simulink model "sampleModel56"  (Simulink 9.1)
settings: Solver=VariableStepAuto  StartTime=0.0  StopTime=10.0  RelTol=1e-3
undefined symbols (not defined in the file): DiscIntNeverNeededParam, Newton, Raphson
libraries: simulink x48
(part 1 of 2)
settings Model: SuppressorTable="22 serialization::archive 11 0 6 0 0 2 8 0 0 0 0 6 0 0 1 0 21 sampleModel56/cfblk75 0 6 0 0 2 8 0 0 0 0 6 41 Simulink:DataType:WarningOverFlowDetected 0 0 0 6 0  0  0 0 0 0 8 20160523 0 0 0 10 57 55 0 1 40 SimulinkFixedPoint:util:Overflowoccurred 0 0 0  0  8 20160523 0 10 57 55 0 1 1 0 21 sampleModel56/cfblk69 2 8 0 41 Simulink:DataType:WarningOverFlowDetected 0 0 0  0  8 20160608 0 15 23 17 0 1 40 SimulinkFixedPoint:util:Overflowoccurred 0 0 0  0  8 20160608 0 15 23 17 0 1"  Creator=DELL  LastModifiedBy=DELL
settings DataIOCC: SaveFormat=Dataset
settings OptimizationCC: LifeSpan=auto
settings DebuggingCC: UnderspecifiedInitializationDetection=Simplified  MergeDetectMultiDrivingBlocksExec=error  SFUnexpectedBacktrackingDiag=error  SFNoUnconditionalDefaultTransitionDiag=error  SFExecutionAtInitializationDiag=warning
settings HardwareCC: ProdBitPerPointer=64  ProdBitPerSizeT=64  ProdBitPerPtrDiffT=64  ProdLargestAtomicFloat=Float  ProdIntDivRoundTo=Zero  ProdEndianess=LittleEndian  ProdWordSize=64  ProdHWDeviceType=Intel->x86-64 (Windows64)
settings ModelReferenceCC: PropagateSignalLabelsOutOfModel=on
settings CodeAppCC: StateflowObjectComments=off
settings GRTTargetCC: TargetLangStandard=C99 (ISO)  CombineOutputUpdateFcns=on  GRTInterface=off
settings ConfigComp: CovMetricSettings=dwe  CovHtmlReporting=off  CovSaveCumulativeToWorkspaceVar=off  CovSaveSingleToWorkspaceVar=off  CovExternalEMLEnable=on

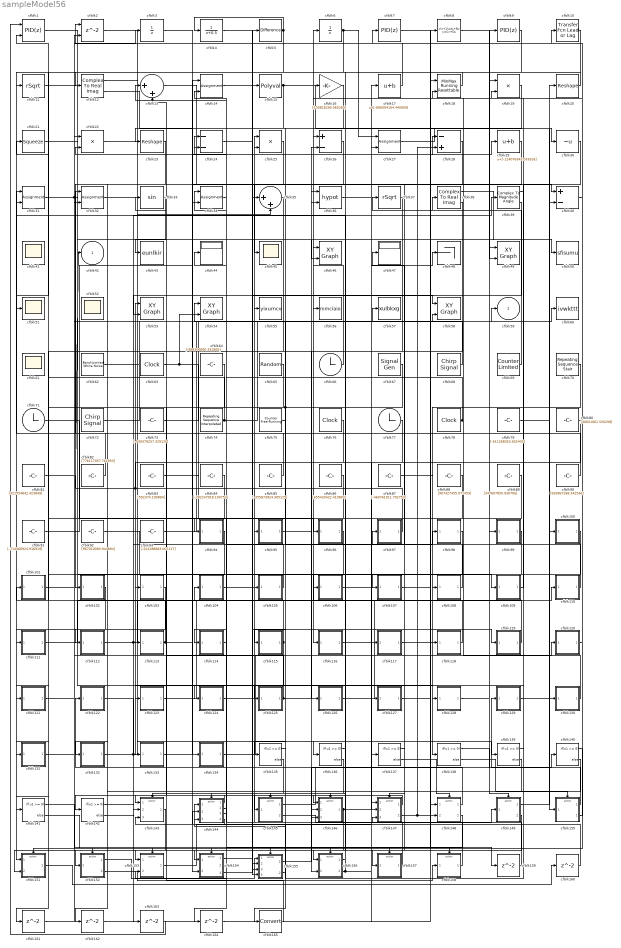
== system sampleModel56 ==
  cfblk1 : simulink/Continuous/PID Controller (2DOF)  Controller=PID  TimeDomain=Discrete-time  SampleTime=1  IntegratorMethod=Forward Euler  FilterMethod=Forward Euler  Form=Parallel  UseFilter=on  ControllerParametersSource=internal  P=1  I=1  D=0  N=100  b=1  c=1  InitialConditionSource=internal  InitialConditionForIntegrator=0  InitialConditionForFilter=0  ExternalReset=none  LimitOutput=off  UpperSaturationLimit=inf  LowerSaturationLimit=-inf  LinearizeAsGain=off  AntiWindupMode=none  Kb=1  TrackingMode=off  Kt=1  PParamMin=[]  PParamMax=[]  IParamMin=[]  IParamMax=[]  DParamMin=[]  DParamMax=[]  NParamMin=[]  NParamMax=[]  bParamMin=[]  bParamMax=[]  cParamMin=[]  cParamMax=[]  KbParamMin=[]  KbParamMax=[]  KtParamMin=[]  KtParamMax=[]  POutMin=[]  POutMax=[]  IOutMin=[]  IOutMax=[]  DOutMin=[]  DOutMax=[]  NOutMin=[]  NOutMax=[]  bOutMin=[]  bOutMax=[]  cOutMin=[]  cOutMax=[]  KbOutMin=[]  KbOutMax=[]  KtOutMin=[]  KtOutMax=[]  IntegratorOutMin=[]  IntegratorOutMax=[]  FilterOutMin=[]  FilterOutMax=[]  SumOutMin=[]  SumOutMax=[]  Sum1OutMin=[]  Sum1OutMax=[]  Sum2OutMin=[]  Sum2OutMax=[]  Sum3OutMin=[]  Sum3OutMax=[]  SumI1OutMin=[]  SumI1OutMax=[]  SumI2OutMin=[]  SumI2OutMax=[]  SumI3OutMin=[]  SumI3OutMax=[]  SumDOutMin=[]  SumDOutMax=[]  SaturationOutMin=[]  SaturationOutMax=[]  IntegratorContinuousStateAttributes=''  IntegratorStateMustResolveToSignalObject=off  IntegratorRTWStateStorageClass=Auto  FilterContinuousStateAttributes=''  FilterStateMustResolveToSignalObject=off  FilterRTWStateStorageClass=Auto  DifferentiatorICPrevScaledInput=0  DifferentiatorOutMin=[]  DifferentiatorOutMax=[]  FilterDiffOutCoefMin=[]  FilterDiffOutCoefMax=[]  SumDenOutMin=[]  SumDenOutMax=[]  SumNumOutMin=[]  SumNumOutMax=[]  ReciprocalOutMin=[]  ReciprocalOutMax=[]  DivideOutMin=[]  DivideOutMax=[]  TunerSelectOption=Transfer Function Based (PID Tuner App)
  cfblk10 : simulink/Discrete/Transfer Fcn Lead or Lag  PoleZ=0.95  ZeroZ=0.75  ICPrevOutput=0.0  ICPrevInput=0.0  DoSatur=off
      settings: SourceProductName=Simulink  SourceProductBaseCode=SL
  cfblk100 : Subsystem
  cfblk101 : Subsystem
  cfblk102 : Subsystem
  cfblk103 : Subsystem
  cfblk104 : Subsystem
  cfblk105 : Subsystem
  cfblk106 : Subsystem
  cfblk107 : Subsystem
  cfblk108 : Subsystem
  cfblk109 : Subsystem
  cfblk11 : Sqrt  Operator=rSqrt  AlgorithmType=Newton-Raphson  SaturateOnIntegerOverflow=on
  cfblk110 : Subsystem
  cfblk111 : Subsystem
  cfblk112 : Subsystem
  cfblk113 : Subsystem
  cfblk114 : Subsystem
  cfblk115 : Subsystem
  cfblk116 : Subsystem
  cfblk117 : Subsystem
  cfblk118 : Subsystem
  cfblk119 : Subsystem
  cfblk12 : ComplexToRealImag
  cfblk120 : Subsystem
  cfblk121 : Subsystem
  cfblk122 : Subsystem
  cfblk123 : Subsystem
  cfblk124 : Subsystem
  cfblk125 : Subsystem
  cfblk126 : Subsystem
  cfblk127 : Subsystem
  cfblk128 : Subsystem
  cfblk129 : Subsystem
  cfblk13 : Sum  Inputs=|++
  cfblk130 : Subsystem
  cfblk131 : Subsystem
  cfblk132 : Subsystem
  cfblk133 : Subsystem
  cfblk134 : Subsystem
  cfblk{135..142} (8 alike) : If  IfExpression=u1 >= 0  SampleTime=1
  cfblk{14,27,31..32,34} (5 alike) : Assignment  DiagnosticForDimensions=Warning  IndexOptions=Index vector (dialog)  Indices=1  OutputSizes=1
  cfblk143 : Subsystem  TreatAsAtomicUnit=on
  cfblk144 : Subsystem  TreatAsAtomicUnit=on
  cfblk145 : Subsystem  TreatAsAtomicUnit=on
  cfblk146 : Subsystem  TreatAsAtomicUnit=on
  cfblk147 : Subsystem  TreatAsAtomicUnit=on
  cfblk148 : Subsystem  TreatAsAtomicUnit=on
  cfblk149 : Subsystem  TreatAsAtomicUnit=on
  cfblk15 : Polyval  Coefs=[ +2.081618890e-019, -1.441693666e-014, +4.719686976e-010, -8.536869453e-006, +1.621573104e-001, -8.087801117e+001 ]
  cfblk150 : Subsystem  TreatAsAtomicUnit=on
  cfblk151 : Subsystem  TreatAsAtomicUnit=on
  cfblk152 : Subsystem  TreatAsAtomicUnit=on
  cfblk153 : Subsystem  TreatAsAtomicUnit=on
  cfblk154 : Subsystem  TreatAsAtomicUnit=on
  cfblk155 : Subsystem  TreatAsAtomicUnit=on
  cfblk156 : Subsystem  TreatAsAtomicUnit=on
  cfblk157 : Subsystem  TreatAsAtomicUnit=on
  cfblk158 : Subsystem  TreatAsAtomicUnit=on
  cfblk{159..164} (6 alike) : Delay  SampleTime=1
  cfblk16 : Gain  Gain=[130818295.065280]
  cfblk165 : DataTypeConversion
  cfblk17 : Bias  Bias=[-890094164.440905]
  cfblk18 : simulink/Math Operations/MinMax Running Resettable  Function=min  vinit=0.0
  cfblk19 : Product
  cfblk2 : Delay  ShowEnablePort=on  SampleTime=1
      settings: InputPortMap=u0,e6
  cfblk20 : Reshape
  cfblk21 : Squeeze
  cfblk22 : Product  Inputs=**
  cfblk23 : Reshape
  cfblk24 : Sum  Inputs=--
  cfblk25 : Product  Inputs=**
  cfblk26 : Sum  Inputs=+-
  cfblk28 : Sum  Inputs=-+
  cfblk29 : Bias  Bias=[-124076343.033326]
  cfblk3 : UnitDelay
  cfblk30 : UnaryMinus
  cfblk33 : Trigonometry
  cfblk35 : Sum  Inputs=|++
  cfblk36 : Math  Operator=hypot  SaturateOnIntegerOverflow=on
  cfblk37 : Sqrt  Operator=rSqrt  AlgorithmType=Newton-Raphson  SaturateOnIntegerOverflow=on
  cfblk38 : ComplexToRealImag
  cfblk39 : ComplexToMagnitudeAngle
  cfblk4 : DiscreteTransferFcn  SampleTime=1
  cfblk40 : Sum  Inputs=+-
  cfblk{41,45,51..52,61} (5 alike) : Scope
      cfblk41 settings: Floating=on
      cfblk52 settings: Floating=on
      cfblk61 settings: Floating=on
  cfblk43 : ToWorkspace  VariableName=eunlkir  SaveFormat=Timeseries  SampleTime=-1
  cfblk44 : Display
  cfblk{46,49,53..54,58} (5 alike) : simulink/Sinks/XY Graph  xmin=-1  xmax=1  ymin=-1  ymax=1  st=-1
  cfblk47 : Display
  cfblk48 : Terminator
  cfblk5 : simulink/Discrete/Difference  ICPrevInput=0.0  OutMin=[]  OutMax=[]  OutDataTypeStr=Inherit: Inherit via back propagation  OutDataType=fixdt(1, 16)  OutScaling=2^-10  DoSatur=off
  cfblk50 : ToWorkspace  VariableName=sfisumu  SaveFormat=Timeseries  SampleTime=-1
  cfblk55 : ToWorkspace  VariableName=yixumcv  SaveFormat=Timeseries  SampleTime=-1
  cfblk56 : ToWorkspace  VariableName=mmciaio  SaveFormat=Timeseries  SampleTime=-1
  cfblk57 : ToWorkspace  VariableName=xulbkxg  SaveFormat=Timeseries  SampleTime=-1
  cfblk6 : UnitDelay
  cfblk60 : ToWorkspace  VariableName=ivwkttt  SaveFormat=Timeseries  SampleTime=-1
  cfblk62 : simulink/Sources/Band-Limited White Noise  Cov=[1765669451.498084]  Ts=0.1  seed=[9360864927.000000]
  cfblk63 : DigitalClock
  cfblk64 : Constant  Value=[-898306890.331865]  SampleTime=1
  cfblk65 : UniformRandomNumber  Minimum=[-2929177195.008087]  Maximum=[2486126280.985762]  Seed=[75996113.000000]  SampleTime=0.1
  cfblk66 : Clock
  cfblk67 : SignalGenerator  WaveForm=square  Amplitude=[871101075.158705]
  cfblk68 : simulink/Sources/Chirp Signal  f1=[-436006107.208133]  T=[-770383043.946067]  f2=[-712322538.075546]
  cfblk69 : simulink/Sources/Counter Limited  uplimit=[311.000000]  tsamp=-1
  cfblk7 : simulink/Continuous/PID Controller  Controller=PID  TimeDomain=Discrete-time  SampleTime=1  IntegratorMethod=Forward Euler  FilterMethod=Forward Euler  Form=Parallel  UseFilter=on  ControllerParametersSource=internal  P=1  I=1  D=0  N=100  InitialConditionSource=internal  InitialConditionForIntegrator=0  InitialConditionForFilter=0  ExternalReset=none  LimitOutput=off  UpperSaturationLimit=inf  LowerSaturationLimit=-inf  LinearizeAsGain=off  AntiWindupMode=none  Kb=1  TrackingMode=off  Kt=1  PParamMin=[]  PParamMax=[]  IParamMin=[]  IParamMax=[]  DParamMin=[]  DParamMax=[]  NParamMin=[]  NParamMax=[]  KbParamMin=[]  KbParamMax=[]  KtParamMin=[]  KtParamMax=[]  POutMin=[]  POutMax=[]  IOutMin=[]  IOutMax=[]  DOutMin=[]  DOutMax=[]  NOutMin=[]  NOutMax=[]  KbOutMin=[]  KbOutMax=[]  KtOutMin=[]  KtOutMax=[]  IntegratorOutMin=[]  IntegratorOutMax=[]  FilterOutMin=[]  FilterOutMax=[]  SumOutMin=[]  SumOutMax=[]  SumI1OutMin=[]  SumI1OutMax=[]  SumI2OutMin=[]  SumI2OutMax=[]  SumI3OutMin=[]  SumI3OutMax=[]  SumDOutMin=[]  SumDOutMax=[]  SaturationOutMin=[]  SaturationOutMax=[]  IntegratorContinuousStateAttributes=''  IntegratorStateMustResolveToSignalObject=off  IntegratorRTWStateStorageClass=Auto  FilterContinuousStateAttributes=''  FilterStateMustResolveToSignalObject=off  FilterRTWStateStorageClass=Auto  DifferentiatorICPrevScaledInput=0  DifferentiatorOutMin=[]  DifferentiatorOutMax=[]  FilterDiffOutCoefMin=[]  FilterDiffOutCoefMax=[]  SumDenOutMin=[]  SumDenOutMax=[]  SumNumOutMin=[]  SumNumOutMax=[]  ReciprocalOutMin=[]  ReciprocalOutMax=[]  DivideOutMin=[]  DivideOutMax=[]  TunerSelectOption=Transfer Function Based (PID Tuner App)
  cfblk70 : simulink/Sources/Repeating Sequence Stair  OutValues=[-137778962.347903, -933746731.009495]  tsamp=-1  OutMin=[]  OutMax=[]  OutDataTypeStr=double  OutputDataTypeScalingMode=double  OutDataType=fixdt(0,8)  ConRadixGroup=Best Precision: Vector-wise  OutScaling=2^-12
  cfblk71 : Clock
  cfblk72 : simulink/Sources/Chirp Signal  f1=[607713325.330179]  T=[-397967056.037934]  f2=[-322334761.817164]
  cfblk73 : Constant  Value=[-939379257.329126]  SampleTime=1
  cfblk74 : simulink/Sources/Repeating Sequence Interpolated  OutValues=[-450364325.771331, -592291030.107568, 415883550.451859, -474150290.301098, 743512600.610433]  TimeValues=[0 0.1 0.5 0.6 1].'  LookUpMeth=Interpolation-Use End Values  tsamp=0.01  OutMin=[]  OutMax=[]  OutDataTypeStr=double  OutputDataTypeScalingMode=double  OutDataType=fixdt(0,8)  OutScaling=2^-10
  cfblk75 : simulink/Sources/Counter Free-Running  NumBits=[38.000000]  tsamp=-1
  cfblk76 : DigitalClock
  cfblk77 : Clock
  cfblk78 : DigitalClock
  cfblk79 : Constant  Value=[-611268353.652435]  SampleTime=1
  cfblk8 : DiscreteStateSpace
  cfblk80 : Constant  Value=[30601061.526258]  SampleTime=1
  cfblk81 : Constant  Value=[321554842.423849]  SampleTime=1
  cfblk82 : Constant  Value=[776117057.761953]  SampleTime=1
  cfblk83 : Constant  Value=[592374.190894]  SampleTime=1
  cfblk84 : Constant  Value=[-282247918.100753]  SampleTime=1
  cfblk85 : Constant  Value=[-355873924.305125]  SampleTime=1
  cfblk86 : Constant  Value=[655420422.410893]  SampleTime=1
  cfblk87 : Constant  Value=[-460761911.792753]  SampleTime=1
  cfblk88 : Constant  Value=[907427455.071453]  SampleTime=1
  cfblk89 : Constant  Value=[347607850.930706]  SampleTime=1
  cfblk9 : simulink/Continuous/PID Controller  Controller=PID  TimeDomain=Discrete-time  SampleTime=1  IntegratorMethod=Forward Euler  FilterMethod=Forward Euler  Form=Parallel  UseFilter=on  ControllerParametersSource=internal  P=1  I=1  D=0  N=100  InitialConditionSource=internal  InitialConditionForIntegrator=0  InitialConditionForFilter=0  ExternalReset=none  LimitOutput=off  UpperSaturationLimit=inf  LowerSaturationLimit=-inf  LinearizeAsGain=off  AntiWindupMode=none  Kb=1  TrackingMode=off  Kt=1  PParamMin=[]  PParamMax=[]  IParamMin=[]  IParamMax=[]  DParamMin=[]  DParamMax=[]  NParamMin=[]  NParamMax=[]  KbParamMin=[]  KbParamMax=[]  KtParamMin=[]  KtParamMax=[]  POutMin=[]  POutMax=[]  IOutMin=[]  IOutMax=[]  DOutMin=[]  DOutMax=[]  NOutMin=[]  NOutMax=[]  KbOutMin=[]  KbOutMax=[]  KtOutMin=[]  KtOutMax=[]  IntegratorOutMin=[]  IntegratorOutMax=[]  FilterOutMin=[]  FilterOutMax=[]  SumOutMin=[]  SumOutMax=[]  SumI1OutMin=[]  SumI1OutMax=[]  SumI2OutMin=[]  SumI2OutMax=[]  SumI3OutMin=[]  SumI3OutMax=[]  SumDOutMin=[]  SumDOutMax=[]  SaturationOutMin=[]  SaturationOutMax=[]  IntegratorContinuousStateAttributes=''  IntegratorStateMustResolveToSignalObject=off  IntegratorRTWStateStorageClass=Auto  FilterContinuousStateAttributes=''  FilterStateMustResolveToSignalObject=off  FilterRTWStateStorageClass=Auto  DifferentiatorICPrevScaledInput=0  DifferentiatorOutMin=[]  DifferentiatorOutMax=[]  FilterDiffOutCoefMin=[]  FilterDiffOutCoefMax=[]  SumDenOutMin=[]  SumDenOutMax=[]  SumNumOutMin=[]  SumNumOutMax=[]  ReciprocalOutMin=[]  ReciprocalOutMax=[]  DivideOutMin=[]  DivideOutMax=[]  TunerSelectOption=Transfer Function Based (PID Tuner App)
  cfblk90 : Constant  Value=[926967268.342546]  SampleTime=1
  cfblk91 : Constant  Value=[-714366924.916919]  SampleTime=1
  cfblk92 : Constant  Value=[967010083.944894]  SampleTime=1
  cfblk93 : Constant  Value=[-524188683.007117]  SampleTime=1
  cfblk94 : Subsystem
  cfblk95 : Subsystem
  cfblk96 : Subsystem
  cfblk97 : Subsystem
  cfblk98 : Subsystem
  cfblk99 : Subsystem
  cfblk42 : Outport
  cfblk59 : Outport  Port=2
  wires:
  cfblk148/1(cfblk2) -> cfblk122/1(cfblk1)
  cfblk119/1(cfblk2) -> cfblk6/1
  cfblk12/1 -> cfblk96/1(cfblk1)
  cfblk132/1(cfblk2) -> cfblk136/1, cfblk98/1(cfblk1)
  cfblk158/1(cfblk2) -> cfblk25/1
  cfblk1/1 -> cfblk147/1(cfblk1)
  cfblk121/1(cfblk2) -> cfblk57/1
  cfblk30/1 -> cfblk144/1(cfblk1)
  cfblk126/1(cfblk2) -> cfblk110/1(cfblk1)
  cfblk154/1(cfblk2) -> cfblk5/1
  cfblk157/1(cfblk2) -> cfblk34/1
  cfblk102/1(cfblk2) -> cfblk151/1(cfblk1)
  cfblk5/1 -> cfblk4/1, cfblk34/2
  cfblk21/1 -> cfblk138/1
  cfblk69/1 -> cfblk37/1
  cfblk104/1(cfblk2) -> cfblk95/1(cfblk1)
  cfblk91/1 -> cfblk14/1
  cfblk85/1 -> cfblk25/2
  cfblk28/1 -> cfblk45/1
  cfblk27/1 -> cfblk30/1
  cfblk62/1 -> cfblk15/1
  cfblk120/1(cfblk2) -> cfblk7/1
  cfblk99/1(cfblk2) -> cfblk116/1(cfblk1)
  cfblk36/1 -> cfblk17/1
  cfblk129/1(cfblk2) -> cfblk20/1
  cfblk146/1(cfblk2) -> cfblk59/1, cfblk155/4(cfblk13)
  cfblk156/1(cfblk2) -> cfblk56/1
  cfblk66/1 -> cfblk46/1
  cfblk23/1 -> cfblk102/1(cfblk1)
  cfblk14/1 -> cfblk119/1(cfblk1)
  cfblk83/1 -> cfblk126/1(cfblk1)
  cfblk112/1(cfblk2) -> cfblk104/1(cfblk1), cfblk39/1
  cfblk13/1 -> cfblk105/1(cfblk1)
  cfblk108/1(cfblk2) -> cfblk55/1
  cfblk87/1 -> cfblk128/1(cfblk1)
  cfblk68/1 -> cfblk54/1
  cfblk98/1(cfblk2) -> cfblk156/1(cfblk1)
  cfblk84/1 -> cfblk133/1(cfblk1)
  cfblk156/2(cfblk14) -> cfblk117/1(cfblk1), cfblk31/2
  cfblk2/1 -> cfblk107/1(cfblk1)
  cfblk31/1 -> cfblk46/2, cfblk3/1
  cfblk123/1(cfblk2) -> cfblk49/1
  cfblk63/1 -> cfblk156/2(cfblk13), cfblk54/2
  cfblk145/1(cfblk2) -> cfblk19/1
  cfblk93/1 -> cfblk35/1
  cfblk80/1 -> cfblk147/2(cfblk15)
  cfblk153/1(cfblk2) -> cfblk127/1(cfblk1)
  cfblk10/1 -> cfblk146/1(cfblk1)
  cfblk32/1 -> cfblk148/1(cfblk1)
  cfblk11/1 -> cfblk134/1(cfblk1)
  cfblk6/1 -> cfblk111/1(cfblk1), cfblk27/1
  cfblk89/1 -> cfblk124/1(cfblk1)
  cfblk110/1(cfblk2) -> cfblk47/1
  cfblk70/1 -> cfblk108/1(cfblk1)
  cfblk17/1 -> cfblk2/1
  cfblk33/1 -> cfblk43/1
  cfblk90/1 -> cfblk31/1
  cfblk114/1(cfblk2) -> cfblk154/1(cfblk1)
  cfblk71/1 -> cfblk94/1(cfblk1)
  cfblk20/1 -> cfblk11/1
  cfblk130/1(cfblk2) -> cfblk38/1
  cfblk64/1 -> cfblk132/1(cfblk1)
  cfblk96/1(cfblk2) -> cfblk114/1(cfblk1)
  cfblk113/1(cfblk2) -> cfblk97/1(cfblk1), cfblk1/2
  cfblk29/1 -> cfblk157/1(cfblk1)
  cfblk78/1 -> cfblk24/1, cfblk18/2
  cfblk79/1 -> cfblk130/1(cfblk1)
  cfblk18/1 -> cfblk12/1
  cfblk73/1 -> cfblk60/1
  cfblk109/1(cfblk2) -> cfblk19/2
  cfblk94/1(cfblk2) -> cfblk131/1(cfblk1)
  cfblk40/1 -> cfblk10/1
  cfblk133/1(cfblk2) -> cfblk26/1
  cfblk111/1(cfblk2) -> cfblk36/1
  cfblk37/1 -> cfblk146/2(cfblk6)
  cfblk3/1 -> cfblk40/1
  cfblk125/1(cfblk2) -> cfblk36/2, cfblk13/2
  cfblk149/1(cfblk2) -> cfblk40/2
  cfblk15/1 -> cfblk100/1(cfblk1), cfblk155/3(cfblk12)
  cfblk19/1 -> cfblk115/1(cfblk1)
  cfblk115/1(cfblk2) -> cfblk143/1(cfblk1), cfblk101/1(cfblk1)
  cfblk26/1 -> cfblk152/1(cfblk1)
  cfblk100/1(cfblk2) -> cfblk145/1(cfblk1)
  cfblk8/1 -> cfblk49/2
  cfblk72/1 -> cfblk9/1
  cfblk77/1 -> cfblk103/1(cfblk1)
  cfblk103/1(cfblk2) -> cfblk112/1(cfblk1)
  cfblk128/1(cfblk2) -> cfblk99/1(cfblk1)
  cfblk147/1(cfblk2) -> cfblk142/1
  cfblk86/1 -> cfblk141/1
  cfblk82/1 -> cfblk32/1
  cfblk127/1(cfblk2) -> cfblk8/1
  cfblk65/1 -> cfblk113/1(cfblk1)
  cfblk22/1 -> cfblk35/2
  cfblk149/2(cfblk12) -> cfblk153/1(cfblk1)
  cfblk92/1 -> cfblk106/1(cfblk1)
  cfblk131/1(cfblk2) -> cfblk120/1(cfblk1)
  cfblk124/1(cfblk2) -> cfblk18/1
  cfblk118/1(cfblk2) -> cfblk24/2
  cfblk24/1 -> cfblk58/1
  cfblk150/1(cfblk2) -> cfblk129/1(cfblk1)
  cfblk16/1 -> cfblk23/1
  cfblk9/1 -> cfblk51/1
  cfblk74/1 -> cfblk21/1, cfblk27/2
  cfblk105/1(cfblk2) -> cfblk44/1
  cfblk38/1 -> cfblk150/1(cfblk1)
  cfblk95/1(cfblk2) -> cfblk109/1(cfblk1)
  cfblk34/1 -> cfblk14/2
  cfblk134/1(cfblk2) -> cfblk26/2
  cfblk143/1(cfblk2) -> cfblk151/2(cfblk8)
  cfblk150/2(cfblk8) -> cfblk16/1
  cfblk116/1(cfblk2) -> cfblk48/1
  cfblk101/1(cfblk2) -> cfblk32/2
  cfblk145/2(cfblk16) -> cfblk149/1(cfblk1)
  cfblk152/1(cfblk2) -> cfblk155/1(cfblk1)
  cfblk4/1 -> cfblk50/1
  cfblk7/1 -> cfblk139/1
  cfblk106/1(cfblk2) -> cfblk58/2
  cfblk144/1(cfblk2) -> cfblk143/2(cfblk8)
  cfblk67/1 -> cfblk121/1(cfblk1), cfblk135/1
  cfblk76/1 -> cfblk123/1(cfblk1)
  cfblk152/2(cfblk10) -> cfblk158/1(cfblk1)
  cfblk144/2(cfblk15) -> cfblk13/1
  cfblk39/1 -> cfblk125/1(cfblk1)
  cfblk144/3(cfblk16) -> cfblk22/2
  cfblk88/1 -> cfblk146/3(cfblk7)
  cfblk147/2(cfblk17) -> cfblk29/1, cfblk28/2
  cfblk144/4(cfblk17) -> cfblk143/3(cfblk9)
  cfblk117/1(cfblk2) -> cfblk118/1(cfblk1)
  cfblk97/1(cfblk2) -> cfblk53/1, cfblk42/1
  cfblk155/1(cfblk2) -> cfblk140/1
  cfblk154/2(cfblk16) -> cfblk153/2(cfblk13)
  cfblk81/1 -> cfblk2/2
  cfblk38/2 -> cfblk155/2(cfblk11)
  cfblk39/2 -> cfblk53/2
  cfblk155/2(cfblk14) -> cfblk144/3(cfblk14)
  cfblk154/3(cfblk17) -> cfblk28/1
  cfblk12/2 -> cfblk154/2(cfblk15)
  cfblk135/1 -> cfblk143/Action
  cfblk135/2 -> cfblk144/Action
  cfblk136/1 -> cfblk145/Action
  cfblk136/2 -> cfblk146/Action
  cfblk137/1 -> cfblk147/Action
  cfblk137/2 -> cfblk148/Action
  cfblk138/1 -> cfblk149/Action
  cfblk138/2 -> cfblk150/Action
  cfblk139/1 -> cfblk151/Action
  cfblk139/2 -> cfblk152/Action
  cfblk140/1 -> cfblk153/Action
  cfblk140/2 -> cfblk154/Action
  cfblk141/1 -> cfblk155/Action
  cfblk141/2 -> cfblk156/Action
  cfblk142/1 -> cfblk157/Action
  cfblk142/2 -> cfblk158/Action
  cfblk107/1(cfblk2) -> cfblk159/1
  cfblk159/1 -> cfblk147/3(cfblk16)
  cfblk151/1(cfblk2) -> cfblk160/1
  cfblk160/1 -> cfblk144/2(cfblk13)
  cfblk35/1 -> cfblk161/1
  cfblk161/1 -> cfblk22/1
  cfblk25/1 -> cfblk162/1
  cfblk162/1 -> cfblk148/2(cfblk14)
  cfblk122/1(cfblk2) -> cfblk163/1
  cfblk163/1 -> cfblk1/1
  cfblk148/2(cfblk15) -> cfblk164/1
  cfblk164/1 -> cfblk137/1
  cfblk75/1 -> cfblk165/1
  cfblk165/1 -> cfblk33/1

== system sampleModel56/cfblk100 ==
  cfblk1 : Inport
  cfblk2 : Outport
  wires:
  cfblk1/1 -> cfblk2/1

== system sampleModel56/cfblk101 ==
  cfblk1 : Inport
  cfblk2 : Outport
  wires:
  cfblk1/1 -> cfblk2/1

== system sampleModel56/cfblk102 ==
  cfblk1 : Inport
  cfblk2 : Outport
  wires:
  cfblk1/1 -> cfblk2/1

== system sampleModel56/cfblk103 ==
  cfblk1 : Inport
  cfblk2 : Outport
  wires:
  cfblk1/1 -> cfblk2/1

== system sampleModel56/cfblk104 ==
  cfblk1 : Inport
  cfblk2 : Outport
  wires:
  cfblk1/1 -> cfblk2/1

== system sampleModel56/cfblk105 ==
  cfblk1 : Inport
  cfblk2 : Outport
  wires:
  cfblk1/1 -> cfblk2/1

== system sampleModel56/cfblk106 ==
  cfblk1 : Inport
  cfblk2 : Outport
  wires:
  cfblk1/1 -> cfblk2/1

== system sampleModel56/cfblk107 ==
  cfblk1 : Inport
  cfblk2 : Outport
  wires:
  cfblk1/1 -> cfblk2/1

== system sampleModel56/cfblk108 ==
  cfblk1 : Inport
  cfblk2 : Outport
  wires:
  cfblk1/1 -> cfblk2/1

== system sampleModel56/cfblk109 ==
  cfblk1 : Inport
  cfblk2 : Outport
  wires:
  cfblk1/1 -> cfblk2/1

== system sampleModel56/cfblk110 ==
  cfblk1 : Inport
  cfblk2 : Outport
  wires:
  cfblk1/1 -> cfblk2/1

== system sampleModel56/cfblk111 ==
  cfblk1 : Inport
  cfblk2 : Outport
  wires:
  cfblk1/1 -> cfblk2/1

== system sampleModel56/cfblk112 ==
  cfblk1 : Inport
  cfblk2 : Outport
  wires:
  cfblk1/1 -> cfblk2/1

== system sampleModel56/cfblk113 ==
  cfblk1 : Inport
  cfblk2 : Outport
  wires:
  cfblk1/1 -> cfblk2/1

== system sampleModel56/cfblk114 ==
  cfblk1 : Inport
  cfblk2 : Outport
  wires:
  cfblk1/1 -> cfblk2/1

== system sampleModel56/cfblk115 ==
  cfblk1 : Inport
  cfblk2 : Outport
  wires:
  cfblk1/1 -> cfblk2/1

== system sampleModel56/cfblk116 ==
  cfblk1 : Inport
  cfblk2 : Outport
  wires:
  cfblk1/1 -> cfblk2/1

== system sampleModel56/cfblk117 ==
  cfblk1 : Inport
  cfblk2 : Outport
  wires:
  cfblk1/1 -> cfblk2/1

== system sampleModel56/cfblk118 ==
  cfblk1 : Inport
  cfblk2 : Outport
  wires:
  cfblk1/1 -> cfblk2/1

== system sampleModel56/cfblk119 ==
  cfblk1 : Inport
  cfblk2 : Outport
  wires:
  cfblk1/1 -> cfblk2/1

== system sampleModel56/cfblk120 ==
  cfblk1 : Inport
  cfblk2 : Outport
  wires:
  cfblk1/1 -> cfblk2/1

== system sampleModel56/cfblk121 ==
  cfblk1 : Inport
  cfblk2 : Outport
  wires:
  cfblk1/1 -> cfblk2/1

== system sampleModel56/cfblk122 ==
  cfblk1 : Inport
  cfblk2 : Outport
  wires:
  cfblk1/1 -> cfblk2/1

== system sampleModel56/cfblk123 ==
  cfblk1 : Inport
  cfblk2 : Outport
  wires:
  cfblk1/1 -> cfblk2/1

== system sampleModel56/cfblk124 ==
  cfblk1 : Inport
  cfblk2 : Outport
  wires:
  cfblk1/1 -> cfblk2/1

== system sampleModel56/cfblk125 ==
  cfblk1 : Inport
  cfblk2 : Outport
  wires:
  cfblk1/1 -> cfblk2/1

== system sampleModel56/cfblk126 ==
  cfblk1 : Inport
  cfblk2 : Outport
  wires:
  cfblk1/1 -> cfblk2/1

== system sampleModel56/cfblk127 ==
  cfblk1 : Inport
  cfblk2 : Outport
  wires:
  cfblk1/1 -> cfblk2/1

== system sampleModel56/cfblk128 ==
  cfblk1 : Inport
  cfblk2 : Outport
  wires:
  cfblk1/1 -> cfblk2/1

== system sampleModel56/cfblk129 ==
  cfblk1 : Inport
  cfblk2 : Outport
  wires:
  cfblk1/1 -> cfblk2/1

== system sampleModel56/cfblk130 ==
  cfblk1 : Inport
  cfblk2 : Outport
  wires:
  cfblk1/1 -> cfblk2/1

== system sampleModel56/cfblk131 ==
  cfblk1 : Inport
  cfblk2 : Outport
  wires:
  cfblk1/1 -> cfblk2/1

== system sampleModel56/cfblk132 ==
  cfblk1 : Inport
  cfblk2 : Outport
  wires:
  cfblk1/1 -> cfblk2/1

== system sampleModel56/cfblk133 ==
  cfblk1 : Inport
  cfblk2 : Outport
  wires:
  cfblk1/1 -> cfblk2/1

== system sampleModel56/cfblk134 ==
  cfblk1 : Inport
  cfblk2 : Outport
  wires:
  cfblk1/1 -> cfblk2/1

== system sampleModel56/cfblk143 ==
  cfblk1 : Inport
  cfblk8 : Inport  Port=2
  cfblk9 : Inport  Port=3
  Action Port : ActionPort  ActionType=then
  cfblk10 : Delay
  cfblk3 : simulink/Discrete/Transfer Fcn First Order  PoleZ=0.95  ICPrevOutput=0.0  DoSatur=off
      settings: SourceProductName=Simulink
  cfblk4 : Delay
  cfblk5 : Reshape
  cfblk6 : Sum  Inputs=--
  cfblk7 : Assignment  DiagnosticForDimensions=Warning  IndexOptions=Index vector (dialog)  Indices=1  OutputSizes=1
  cfblk2 : Outport
  wires:
  cfblk5/1 -> cfblk3/1
  cfblk1/1 -> cfblk5/1
  cfblk9/1 -> cfblk2/1
  cfblk8/1 -> cfblk4/1
  cfblk7/1 -> cfblk6/1
  cfblk3/1 -> cfblk7/2
  cfblk4/1 -> cfblk6/2
  cfblk6/1 -> cfblk10/1
  cfblk10/1 -> cfblk7/1

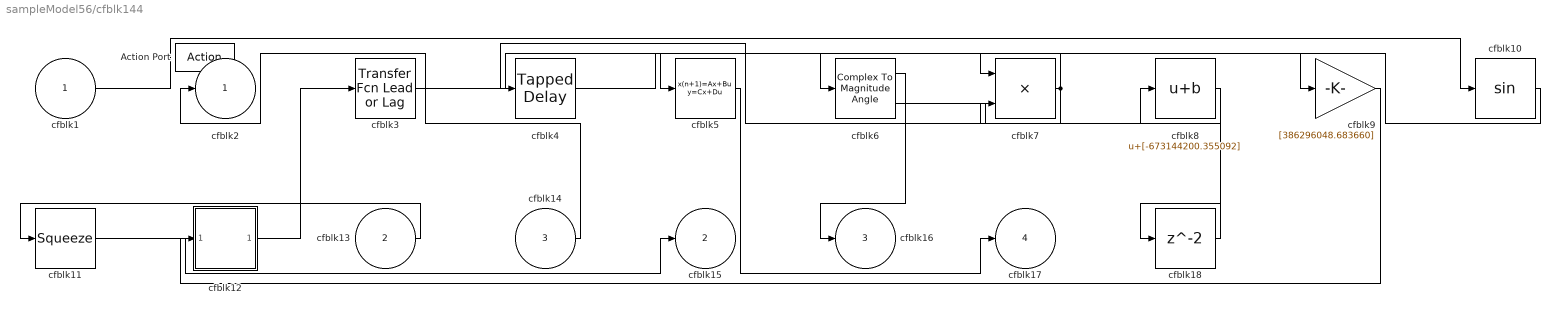
== system sampleModel56/cfblk144 ==
  cfblk1 : Inport
  cfblk13 : Inport  Port=2
  cfblk14 : Inport  Port=3
  Action Port : ActionPort  ActionType=else
  cfblk10 : Trigonometry
  cfblk11 : Squeeze
  cfblk12 : Subsystem
  cfblk18 : Delay
  cfblk3 : simulink/Discrete/Transfer Fcn Lead or Lag  PoleZ=0.95  ZeroZ=0.75  ICPrevOutput=0.0  ICPrevInput=0.0  DoSatur=off
      settings: SourceProductName=Simulink  SourceProductBaseCode=SL
  cfblk4 : simulink/Discrete/Tapped Delay  vinit=0.0  samptime=-1  NumDelays=1  DelayOrder=Oldest  includeCurrent=off
  cfblk5 : DiscreteStateSpace  SampleTime=-1
  cfblk6 : ComplexToMagnitudeAngle
  cfblk7 : Product  Inputs=**
  cfblk8 : Bias  Bias=[-673144200.355092]
  cfblk9 : Gain  Gain=[386296048.683660]
  cfblk2 : Outport
  cfblk15 : Outport  Port=2
  cfblk16 : Outport  Port=3
  cfblk17 : Outport  Port=4
  wires:
  cfblk12/1(cfblk2) -> cfblk3/1
  cfblk11/1 -> cfblk15/1
  cfblk13/1 -> cfblk11/1
  cfblk9/1 -> cfblk12/1(cfblk1)
  cfblk1/1 -> cfblk10/1
  cfblk14/1 -> cfblk2/1
  cfblk3/1 -> cfblk5/1
  cfblk10/1 -> cfblk7/1
  cfblk7/1 -> cfblk4/1, cfblk6/1
  cfblk6/1 -> cfblk16/1
  cfblk6/2 -> cfblk8/1
  cfblk4/1 -> cfblk9/1
  cfblk5/1 -> cfblk17/1
  cfblk8/1 -> cfblk18/1
  cfblk18/1 -> cfblk7/2

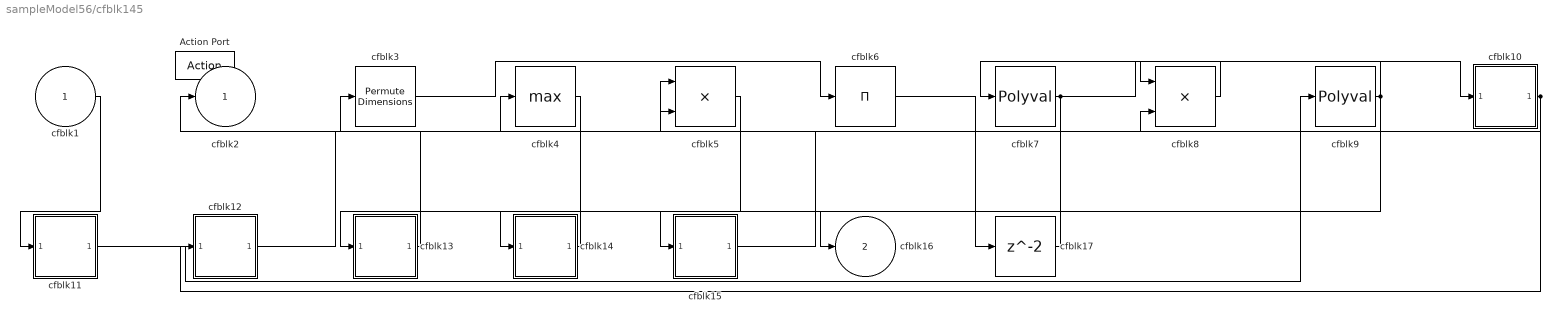
== system sampleModel56/cfblk145 ==
  cfblk1 : Inport
  Action Port : ActionPort  ActionType=then
  cfblk10 : Subsystem
  cfblk11 : Subsystem
  cfblk12 : Subsystem
  cfblk13 : Subsystem
  cfblk14 : Subsystem
  cfblk15 : Subsystem
  cfblk17 : Delay
  cfblk3 : PermuteDimensions
  cfblk4 : MinMax  Function=max
  cfblk5 : Product  Inputs=**
  cfblk6 : Product  Inputs=*
  cfblk7 : Polyval  Coefs=[ +2.081618890e-019, -1.441693666e-014, +4.719686976e-010, -8.536869453e-006, +1.621573104e-001, -8.087801117e+001 ]
  cfblk8 : Product  Inputs=**
  cfblk9 : Polyval  Coefs=[ +2.081618890e-019, -1.441693666e-014, +4.719686976e-010, -8.536869453e-006, +1.621573104e-001, -8.087801117e+001 ]
  cfblk2 : Outport
  cfblk16 : Outport  Port=2
  wires:
  cfblk8/1 -> cfblk7/1
  cfblk13/1(cfblk2) -> cfblk2/1
  cfblk11/1(cfblk2) -> cfblk9/1
  cfblk10/1(cfblk2) -> cfblk12/1(cfblk1), cfblk5/2
  cfblk9/1 -> cfblk8/1, cfblk15/1(cfblk1)
  cfblk4/1 -> cfblk13/1(cfblk1)
  cfblk7/1 -> cfblk16/1, cfblk10/1(cfblk1)
  cfblk1/1 -> cfblk11/1(cfblk1)
  cfblk14/1(cfblk2) -> cfblk4/1
  cfblk3/1 -> cfblk6/1
  cfblk15/1(cfblk2) -> cfblk8/2
  cfblk12/1(cfblk2) -> cfblk5/1
  cfblk5/1 -> cfblk14/1(cfblk1)
  cfblk6/1 -> cfblk17/1
  cfblk17/1 -> cfblk3/1

== system sampleModel56/cfblk146 ==
  cfblk1 : Inport
  cfblk6 : Inport  Port=2
  cfblk7 : Inport  Port=3
  Action Port : ActionPort  ActionType=else
  cfblk10 : Delay
  cfblk3 : simulink/Discrete/Transfer Fcn First Order  PoleZ=0.95  ICPrevOutput=0.0  DoSatur=off
      settings: SourceProductName=Simulink
  cfblk4 : Subsystem
  cfblk5 : If  IfExpression=u1 >= 0  SampleTime=1
  cfblk8 : Subsystem  TreatAsAtomicUnit=on
  cfblk9 : Subsystem  TreatAsAtomicUnit=on
  cfblk2 : Outport
  wires:
  cfblk9/1(cfblk2) -> cfblk2/1
  cfblk8/1(cfblk2) -> cfblk3/1
  cfblk6/1 -> cfblk5/1
  cfblk7/1 -> cfblk8/1(cfblk1)
  cfblk4/1(cfblk2) -> cfblk9/1(cfblk1)
  cfblk5/1 -> cfblk8/Action
  cfblk5/2 -> cfblk9/Action
  cfblk9/2(cfblk9) -> cfblk10/1
  cfblk10/1 -> cfblk4/1(cfblk1)

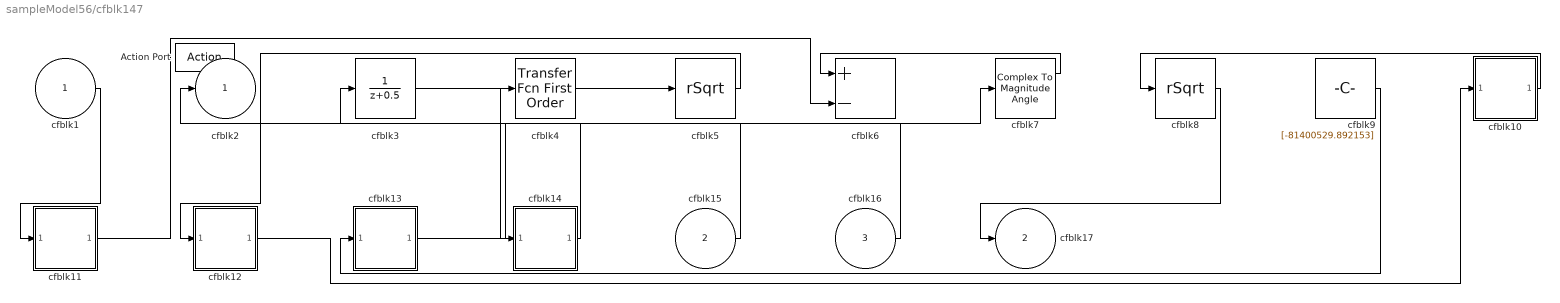
== system sampleModel56/cfblk147 ==
  cfblk1 : Inport
  cfblk15 : Inport  Port=2
  cfblk16 : Inport  Port=3
  Action Port : ActionPort  ActionType=then
  cfblk10 : Subsystem
  cfblk11 : Subsystem
  cfblk12 : Subsystem
  cfblk13 : Subsystem
  cfblk14 : Subsystem
  cfblk3 : DiscreteTransferFcn
  cfblk4 : simulink/Discrete/Transfer Fcn First Order  PoleZ=0.95  ICPrevOutput=0.0  DoSatur=off
      settings: SourceProductName=Simulink
  cfblk5 : Sqrt  Operator=rSqrt  AlgorithmType=Newton-Raphson  SaturateOnIntegerOverflow=on
  cfblk6 : Sum  Inputs=+-
  cfblk7 : ComplexToMagnitudeAngle
  cfblk8 : Sqrt  Operator=rSqrt  AlgorithmType=Newton-Raphson  SaturateOnIntegerOverflow=on
  cfblk9 : Constant  Value=[-81400529.892153]  SampleTime=1
  cfblk2 : Outport
  cfblk17 : Outport  Port=2
  wires:
  cfblk10/1(cfblk2) -> cfblk8/1
  cfblk13/1(cfblk2) -> cfblk7/1
  cfblk1/1 -> cfblk11/1(cfblk1)
  cfblk5/1 -> cfblk12/1(cfblk1)
  cfblk8/1 -> cfblk17/1
  cfblk4/1 -> cfblk5/1
  cfblk3/1 -> cfblk14/1(cfblk1)
  cfblk9/1 -> cfblk13/1(cfblk1)
  cfblk15/1 -> cfblk3/1
  cfblk12/1(cfblk2) -> cfblk10/1(cfblk1)
  cfblk16/1 -> cfblk4/1
  cfblk14/1(cfblk2) -> cfblk2/1
  cfblk7/1 -> cfblk6/1
  cfblk11/1(cfblk2) -> cfblk6/2

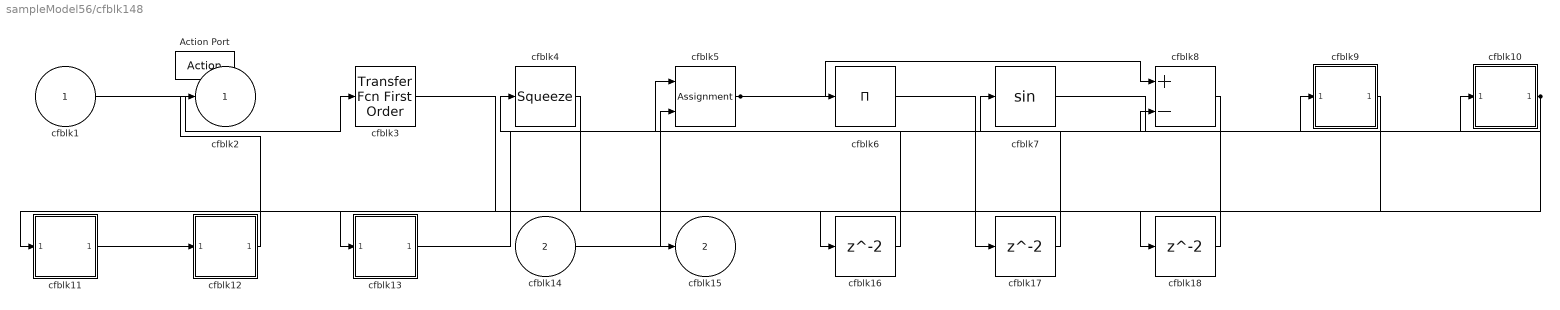
== system sampleModel56/cfblk148 ==
  cfblk1 : Inport
  cfblk14 : Inport  Port=2
  Action Port : ActionPort  ActionType=else
  cfblk10 : Subsystem
  cfblk11 : Subsystem
  cfblk12 : Subsystem
  cfblk13 : Subsystem
  cfblk16 : Delay
  cfblk17 : Delay
  cfblk18 : Delay
  cfblk3 : simulink/Discrete/Transfer Fcn First Order  PoleZ=0.95  ICPrevOutput=0.0  DoSatur=off
      settings: SourceProductName=Simulink
  cfblk4 : Squeeze
  cfblk5 : Assignment  DiagnosticForDimensions=Warning  IndexOptions=Index vector (dialog)  Indices=1  OutputSizes=1
  cfblk6 : Product  Inputs=*
  cfblk7 : Trigonometry
  cfblk8 : Sum  Inputs=+-
  cfblk9 : Subsystem
  cfblk2 : Outport
  cfblk15 : Outport  Port=2
  wires:
  cfblk1/1 -> cfblk3/1
  cfblk13/1(cfblk2) -> cfblk10/1(cfblk1)
  cfblk12/1(cfblk2) -> cfblk2/1
  cfblk5/1 -> cfblk8/1, cfblk6/1
  cfblk7/1 -> cfblk9/1(cfblk1)
  cfblk10/1(cfblk2) -> cfblk8/2, cfblk11/1(cfblk1)
  cfblk11/1(cfblk2) -> cfblk12/1(cfblk1)
  cfblk4/1 -> cfblk13/1(cfblk1)
  cfblk14/1 -> cfblk5/2
  cfblk3/1 -> cfblk15/1
  cfblk8/1 -> cfblk16/1
  cfblk16/1 -> cfblk4/1
  cfblk6/1 -> cfblk17/1
  cfblk17/1 -> cfblk5/1
  cfblk9/1(cfblk2) -> cfblk18/1
  cfblk18/1 -> cfblk7/1

== system sampleModel56/cfblk149 ==
  cfblk1 : Inport
  Action Port : ActionPort  ActionType=then
  cfblk10 : Subsystem
  cfblk11 : Subsystem
  cfblk3 : simulink/Continuous/PID Controller  Controller=PID  TimeDomain=Discrete-time  SampleTime=-1  IntegratorMethod=Forward Euler  FilterMethod=Forward Euler  Form=Parallel  UseFilter=on  ControllerParametersSource=internal  P=1  I=1  D=0  N=100  InitialConditionSource=internal  InitialConditionForIntegrator=0  InitialConditionForFilter=0  ExternalReset=none  LimitOutput=off  UpperSaturationLimit=inf  LowerSaturationLimit=-inf  LinearizeAsGain=off  AntiWindupMode=none  Kb=1  TrackingMode=off  Kt=1  PParamMin=[]  PParamMax=[]  IParamMin=[]  IParamMax=[]  DParamMin=[]  DParamMax=[]  NParamMin=[]  NParamMax=[]  KbParamMin=[]  KbParamMax=[]  KtParamMin=[]  KtParamMax=[]  POutMin=[]  POutMax=[]  IOutMin=[]  IOutMax=[]  DOutMin=[]  DOutMax=[]  NOutMin=[]  NOutMax=[]  KbOutMin=[]  KbOutMax=[]  KtOutMin=[]  KtOutMax=[]  IntegratorOutMin=[]  IntegratorOutMax=[]  FilterOutMin=[]  FilterOutMax=[]  SumOutMin=[]  SumOutMax=[]  SumI1OutMin=[]  SumI1OutMax=[]  SumI2OutMin=[]  SumI2OutMax=[]  SumI3OutMin=[]  SumI3OutMax=[]  SumDOutMin=[]  SumDOutMax=[]  SaturationOutMin=[]  SaturationOutMax=[]  IntegratorContinuousStateAttributes=''  IntegratorStateMustResolveToSignalObject=off  IntegratorRTWStateStorageClass=Auto  FilterContinuousStateAttributes=''  FilterStateMustResolveToSignalObject=off  FilterRTWStateStorageClass=Auto  DifferentiatorICPrevScaledInput=0  DifferentiatorOutMin=[]  DifferentiatorOutMax=[]  FilterDiffOutCoefMin=[]  FilterDiffOutCoefMax=[]  SumDenOutMin=[]  SumDenOutMax=[]  SumNumOutMin=[]  SumNumOutMax=[]  ReciprocalOutMin=[]  ReciprocalOutMax=[]  DivideOutMin=[]  DivideOutMax=[]  TunerSelectOption=Transfer Function Based (PID Tuner App)
  cfblk4 : Trigonometry
  cfblk5 : simulink/Math Operations/MinMax Running Resettable  Function=min  vinit=0.0
  cfblk6 : simulink/Math Operations/MinMax Running Resettable  Function=min  vinit=0.0
  cfblk7 : Sqrt  SaturateOnIntegerOverflow=on
  cfblk8 : Polyval  Coefs=[ +2.081618890e-019, -1.441693666e-014, +4.719686976e-010, -8.536869453e-006, +1.621573104e-001, -8.087801117e+001 ]
  cfblk9 : Subsystem
  cfblk2 : Outport
  cfblk12 : Outport  Port=2
  wires:
  cfblk4/1 -> cfblk12/1
  cfblk6/1 -> cfblk7/1, cfblk5/2
  cfblk11/1(cfblk2) -> cfblk10/1(cfblk1)
  cfblk1/1 -> cfblk8/1
  cfblk8/1 -> cfblk9/1(cfblk1), cfblk6/2
  cfblk5/1 -> cfblk2/1
  cfblk9/1(cfblk2) -> cfblk3/1
  cfblk3/1 -> cfblk11/1(cfblk1)
  cfblk7/1 -> cfblk4/1
  cfblk10/1(cfblk2) -> cfblk6/1, cfblk5/1

== system sampleModel56/cfblk150 ==
  cfblk1 : Inport
  Action Port : ActionPort  ActionType=else
  cfblk10 : Delay
  cfblk3 : simulink/Discrete/Tapped Delay  vinit=0.0  samptime=-1  NumDelays=1  DelayOrder=Oldest  includeCurrent=off
  cfblk4 : MinMax  Function=max  Inputs=2
  cfblk5 : Squeeze
  cfblk6 : Subsystem
  cfblk7 : Subsystem
  cfblk9 : Delay
  cfblk2 : Outport
  cfblk8 : Outport  Port=2
  wires:
  cfblk3/1 -> cfblk5/1
  cfblk1/1 -> cfblk2/1, cfblk7/1(cfblk1), cfblk4/2
  cfblk4/1 -> cfblk6/1(cfblk1)
  cfblk7/1(cfblk2) -> cfblk8/1
  cfblk6/1(cfblk2) -> cfblk9/1
  cfblk9/1 -> cfblk4/1
  cfblk5/1 -> cfblk10/1
  cfblk10/1 -> cfblk3/1

== system sampleModel56/cfblk151 ==
  cfblk1 : Inport
  cfblk8 : Inport  Port=2
  Action Port : ActionPort  ActionType=then
  cfblk3 : simulink/Continuous/PID Controller  Controller=PID  TimeDomain=Discrete-time  SampleTime=-1  IntegratorMethod=Forward Euler  FilterMethod=Forward Euler  Form=Parallel  UseFilter=on  ControllerParametersSource=internal  P=1  I=1  D=0  N=100  InitialConditionSource=internal  InitialConditionForIntegrator=0  InitialConditionForFilter=0  ExternalReset=none  LimitOutput=off  UpperSaturationLimit=inf  LowerSaturationLimit=-inf  LinearizeAsGain=off  AntiWindupMode=none  Kb=1  TrackingMode=off  Kt=1  PParamMin=[]  PParamMax=[]  IParamMin=[]  IParamMax=[]  DParamMin=[]  DParamMax=[]  NParamMin=[]  NParamMax=[]  KbParamMin=[]  KbParamMax=[]  KtParamMin=[]  KtParamMax=[]  POutMin=[]  POutMax=[]  IOutMin=[]  IOutMax=[]  DOutMin=[]  DOutMax=[]  NOutMin=[]  NOutMax=[]  KbOutMin=[]  KbOutMax=[]  KtOutMin=[]  KtOutMax=[]  IntegratorOutMin=[]  IntegratorOutMax=[]  FilterOutMin=[]  FilterOutMax=[]  SumOutMin=[]  SumOutMax=[]  SumI1OutMin=[]  SumI1OutMax=[]  SumI2OutMin=[]  SumI2OutMax=[]  SumI3OutMin=[]  SumI3OutMax=[]  SumDOutMin=[]  SumDOutMax=[]  SaturationOutMin=[]  SaturationOutMax=[]  IntegratorContinuousStateAttributes=''  IntegratorStateMustResolveToSignalObject=off  IntegratorRTWStateStorageClass=Auto  FilterContinuousStateAttributes=''  FilterStateMustResolveToSignalObject=off  FilterRTWStateStorageClass=Auto  DifferentiatorICPrevScaledInput=0  DifferentiatorOutMin=[]  DifferentiatorOutMax=[]  FilterDiffOutCoefMin=[]  FilterDiffOutCoefMax=[]  SumDenOutMin=[]  SumDenOutMax=[]  SumNumOutMin=[]  SumNumOutMax=[]  ReciprocalOutMin=[]  ReciprocalOutMax=[]  DivideOutMin=[]  DivideOutMax=[]  TunerSelectOption=Transfer Function Based (PID Tuner App)
  cfblk4 : simulink/Continuous/PID Controller (2DOF)  Controller=PID  TimeDomain=Discrete-time  SampleTime=-1  IntegratorMethod=Forward Euler  FilterMethod=Forward Euler  Form=Parallel  UseFilter=on  ControllerParametersSource=internal  P=1  I=1  D=0  N=100  b=1  c=1  InitialConditionSource=internal  InitialConditionForIntegrator=0  InitialConditionForFilter=0  ExternalReset=none  LimitOutput=off  UpperSaturationLimit=inf  LowerSaturationLimit=-inf  LinearizeAsGain=off  AntiWindupMode=none  Kb=1  TrackingMode=off  Kt=1  PParamMin=[]  PParamMax=[]  IParamMin=[]  IParamMax=[]  DParamMin=[]  DParamMax=[]  NParamMin=[]  NParamMax=[]  bParamMin=[]  bParamMax=[]  cParamMin=[]  cParamMax=[]  KbParamMin=[]  KbParamMax=[]  KtParamMin=[]  KtParamMax=[]  POutMin=[]  POutMax=[]  IOutMin=[]  IOutMax=[]  DOutMin=[]  DOutMax=[]  NOutMin=[]  NOutMax=[]  bOutMin=[]  bOutMax=[]  cOutMin=[]  cOutMax=[]  KbOutMin=[]  KbOutMax=[]  KtOutMin=[]  KtOutMax=[]  IntegratorOutMin=[]  IntegratorOutMax=[]  FilterOutMin=[]  FilterOutMax=[]  SumOutMin=[]  SumOutMax=[]  Sum1OutMin=[]  Sum1OutMax=[]  Sum2OutMin=[]  Sum2OutMax=[]  Sum3OutMin=[]  Sum3OutMax=[]  SumI1OutMin=[]  SumI1OutMax=[]  SumI2OutMin=[]  SumI2OutMax=[]  SumI3OutMin=[]  SumI3OutMax=[]  SumDOutMin=[]  SumDOutMax=[]  SaturationOutMin=[]  SaturationOutMax=[]  IntegratorContinuousStateAttributes=''  IntegratorStateMustResolveToSignalObject=off  IntegratorRTWStateStorageClass=Auto  FilterContinuousStateAttributes=''  FilterStateMustResolveToSignalObject=off  FilterRTWStateStorageClass=Auto  DifferentiatorICPrevScaledInput=0  DifferentiatorOutMin=[]  DifferentiatorOutMax=[]  FilterDiffOutCoefMin=[]  FilterDiffOutCoefMax=[]  SumDenOutMin=[]  SumDenOutMax=[]  SumNumOutMin=[]  SumNumOutMax=[]  ReciprocalOutMin=[]  ReciprocalOutMax=[]  DivideOutMin=[]  DivideOutMax=[]  TunerSelectOption=Transfer Function Based (PID Tuner App)
  cfblk5 : Squeeze
  cfblk6 : Trigonometry
  cfblk7 : Bias  Bias=[-239528194.623381]
  cfblk9 : Delay
  cfblk2 : Outport
  wires:
  cfblk5/1 -> cfblk6/1
  cfblk8/1 -> cfblk7/1
  cfblk3/1 -> cfblk5/1
  cfblk4/1 -> cfblk3/1
  cfblk7/1 -> cfblk2/1
  cfblk1/1 -> cfblk4/2
  cfblk6/1 -> cfblk9/1
  cfblk9/1 -> cfblk4/1

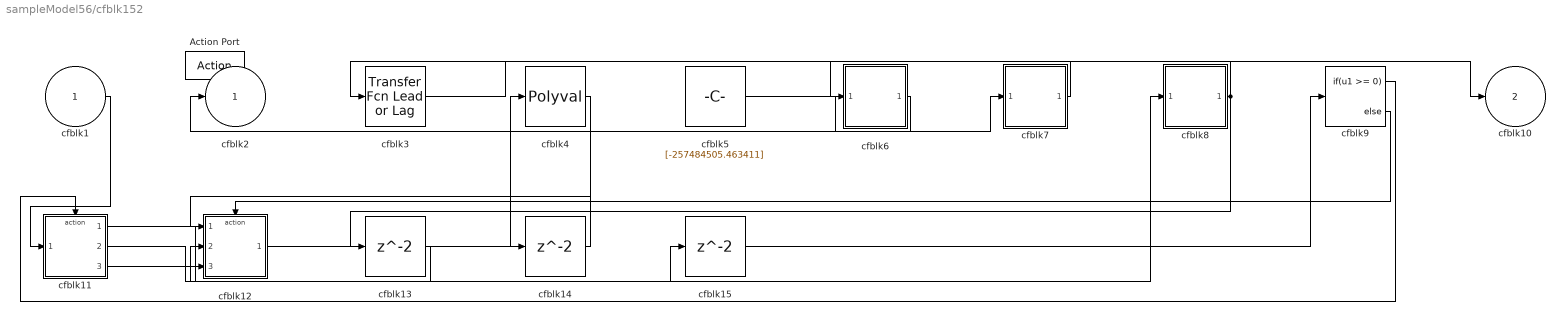
== system sampleModel56/cfblk152 ==
  cfblk1 : Inport
  Action Port : ActionPort  ActionType=else
  cfblk11 : Subsystem  TreatAsAtomicUnit=on
  cfblk12 : Subsystem  TreatAsAtomicUnit=on
  cfblk13 : Delay
  cfblk14 : Delay
  cfblk15 : Delay
  cfblk3 : simulink/Discrete/Transfer Fcn Lead or Lag  PoleZ=0.95  ZeroZ=0.75  ICPrevOutput=0.0  ICPrevInput=0.0  DoSatur=off
      settings: SourceProductName=Simulink  SourceProductBaseCode=SL
  cfblk4 : Polyval  Coefs=[ +2.081618890e-019, -1.441693666e-014, +4.719686976e-010, -8.536869453e-006, +1.621573104e-001, -8.087801117e+001 ]
  cfblk5 : Constant  Value=[-257484505.463411]  SampleTime=1
  cfblk6 : Subsystem
  cfblk7 : Subsystem
  cfblk8 : Subsystem
  cfblk9 : If  IfExpression=u1 >= 0  SampleTime=1
  cfblk2 : Outport
  cfblk10 : Outport  Port=2
  wires:
  cfblk8/1(cfblk2) -> cfblk3/1, cfblk13/1
  cfblk12/1(cfblk2) -> cfblk4/1
  cfblk5/1 -> cfblk7/1(cfblk1)
  cfblk11/1(cfblk2) -> cfblk8/1(cfblk1)
  cfblk1/1 -> cfblk11/1(cfblk1)
  cfblk6/1(cfblk2) -> cfblk2/1
  cfblk3/1 -> cfblk10/1
  cfblk7/1(cfblk2) -> cfblk6/1(cfblk1)
  cfblk11/3(cfblk13) -> cfblk12/2(cfblk9)
  cfblk9/1 -> cfblk11/Action
  cfblk9/2 -> cfblk12/Action
  cfblk13/1 -> cfblk12/3(cfblk10)
  cfblk4/1 -> cfblk14/1
  cfblk14/1 -> cfblk12/1(cfblk1)
  cfblk11/2(cfblk12) -> cfblk15/1
  cfblk15/1 -> cfblk9/1

== system sampleModel56/cfblk153 ==
  cfblk1 : Inport
  cfblk13 : Inport  Port=2
  Action Port : ActionPort  ActionType=then
  cfblk10 : Constant  Value=[796676593.910221]  SampleTime=1
  cfblk11 : Subsystem
  cfblk12 : Subsystem
  cfblk3 : simulink/Discrete/Transfer Fcn Real Zero  ZeroZ=0.75  ICPrevInput=0.0  DoSatur=off
      settings: SourceProductName=Simulink  SourceProductBaseCode=SL
  cfblk4 : Delay
  cfblk5 : simulink/Discrete/Tapped Delay  vinit=0.0  samptime=-1  NumDelays=1  DelayOrder=Oldest  includeCurrent=off
  cfblk6 : simulink/Discrete/Transfer Fcn Lead or Lag  PoleZ=0.95  ZeroZ=0.75  ICPrevOutput=0.0  ICPrevInput=0.0  DoSatur=off
      settings: SourceProductName=Simulink  SourceProductBaseCode=SL
  cfblk7 : simulink/Discrete/Transfer Fcn Real Zero  ZeroZ=0.75  ICPrevInput=0.0  DoSatur=off
      settings: SourceProductName=Simulink  SourceProductBaseCode=SL
  cfblk8 : Sum  Inputs=+
  cfblk9 : Constant  Value=[780818834.997048]  SampleTime=1
  cfblk2 : Outport
  wires:
  cfblk3/1 -> cfblk4/1
  cfblk5/1 -> cfblk6/1
  cfblk8/1 -> cfblk12/1(cfblk1)
  cfblk10/1 -> cfblk5/1
  cfblk12/1(cfblk2) -> cfblk11/1(cfblk1)
  cfblk7/1 -> cfblk2/1
  cfblk1/1 -> cfblk3/1
  cfblk4/1 -> cfblk8/1
  cfblk13/1 -> cfblk7/1

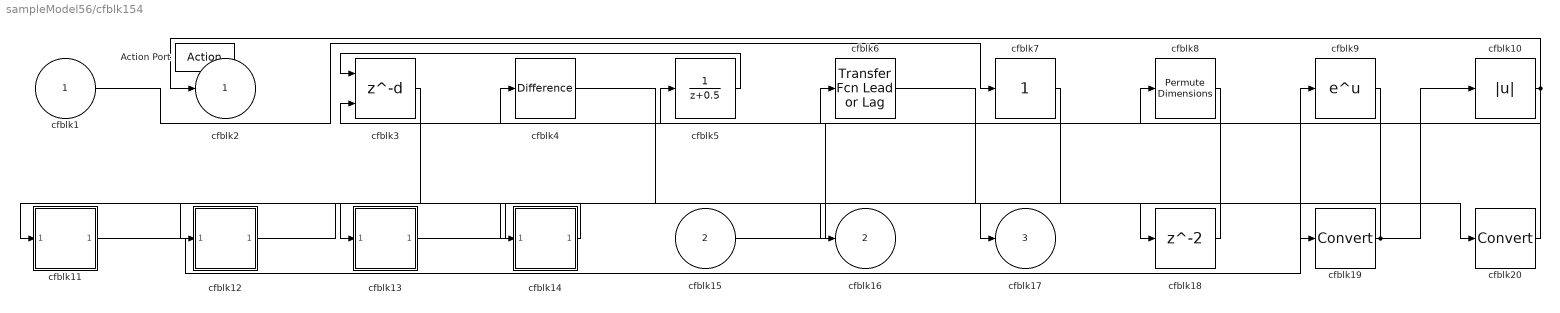
== system sampleModel56/cfblk154 ==
  cfblk1 : Inport
  cfblk15 : Inport  Port=2
  Action Port : ActionPort  ActionType=else
  cfblk10 : Abs
  cfblk11 : Subsystem
  cfblk12 : Subsystem
  cfblk13 : Subsystem
  cfblk14 : Subsystem
  cfblk18 : Delay
  cfblk19 : DataTypeConversion
  cfblk20 : DataTypeConversion
  cfblk3 : Delay  DelayLengthSource=Input port
      settings: InputPortMap=u0,p1
  cfblk4 : simulink/Discrete/Difference  ICPrevInput=0.0  OutMin=[]  OutMax=[]  OutDataTypeStr=Inherit: Inherit via back propagation  OutDataType=fixdt(1, 16)  OutScaling=2^-10  DoSatur=off
  cfblk5 : DiscreteTransferFcn
  cfblk6 : simulink/Discrete/Transfer Fcn Lead or Lag  PoleZ=0.95  ZeroZ=0.75  ICPrevOutput=0.0  ICPrevInput=0.0  DoSatur=off
      settings: SourceProductName=Simulink  SourceProductBaseCode=SL
  cfblk7 : simulink/Math Operations/Slider Gain  gain=1  low=0  high=2
  cfblk8 : PermuteDimensions
  cfblk9 : Math  SaturateOnIntegerOverflow=on
  cfblk2 : Outport
  cfblk16 : Outport  Port=2
  cfblk17 : Outport  Port=3
  wires:
  cfblk13/1(cfblk2) -> cfblk17/1
  cfblk6/1 -> cfblk19/1
  cfblk3/1 -> cfblk11/1(cfblk1)
  cfblk8/1 -> cfblk5/1
  cfblk15/1 -> cfblk8/1
  cfblk11/1(cfblk2) -> cfblk9/1
  cfblk14/1(cfblk2) -> cfblk13/1(cfblk1)
  cfblk7/1 -> cfblk12/1(cfblk1)
  cfblk10/1 -> cfblk2/1, cfblk3/2
  cfblk5/1 -> cfblk3/1
  cfblk9/1 -> cfblk16/1
  cfblk12/1(cfblk2) -> cfblk14/1(cfblk1)
  cfblk1/1 -> cfblk7/1
  cfblk18/1 -> cfblk4/1
  cfblk19/1 -> cfblk18/1, cfblk10/1
  cfblk4/1 -> cfblk20/1
  cfblk20/1 -> cfblk6/1

== system sampleModel56/cfblk155 ==
  cfblk1 : Inport
  cfblk11 : Inport  Port=2
  cfblk12 : Inport  Port=3
  cfblk13 : Inport  Port=4
  Action Port : ActionPort  ActionType=then
  cfblk10 : Subsystem
  cfblk3 : simulink/Continuous/PID Controller  Controller=PID  TimeDomain=Discrete-time  SampleTime=-1  IntegratorMethod=Forward Euler  FilterMethod=Forward Euler  Form=Parallel  UseFilter=on  ControllerParametersSource=internal  P=1  I=1  D=0  N=100  InitialConditionSource=internal  InitialConditionForIntegrator=0  InitialConditionForFilter=0  ExternalReset=none  LimitOutput=off  UpperSaturationLimit=inf  LowerSaturationLimit=-inf  LinearizeAsGain=off  AntiWindupMode=none  Kb=1  TrackingMode=off  Kt=1  PParamMin=[]  PParamMax=[]  IParamMin=[]  IParamMax=[]  DParamMin=[]  DParamMax=[]  NParamMin=[]  NParamMax=[]  KbParamMin=[]  KbParamMax=[]  KtParamMin=[]  KtParamMax=[]  POutMin=[]  POutMax=[]  IOutMin=[]  IOutMax=[]  DOutMin=[]  DOutMax=[]  NOutMin=[]  NOutMax=[]  KbOutMin=[]  KbOutMax=[]  KtOutMin=[]  KtOutMax=[]  IntegratorOutMin=[]  IntegratorOutMax=[]  FilterOutMin=[]  FilterOutMax=[]  SumOutMin=[]  SumOutMax=[]  SumI1OutMin=[]  SumI1OutMax=[]  SumI2OutMin=[]  SumI2OutMax=[]  SumI3OutMin=[]  SumI3OutMax=[]  SumDOutMin=[]  SumDOutMax=[]  SaturationOutMin=[]  SaturationOutMax=[]  IntegratorContinuousStateAttributes=''  IntegratorStateMustResolveToSignalObject=off  IntegratorRTWStateStorageClass=Auto  FilterContinuousStateAttributes=''  FilterStateMustResolveToSignalObject=off  FilterRTWStateStorageClass=Auto  DifferentiatorICPrevScaledInput=0  DifferentiatorOutMin=[]  DifferentiatorOutMax=[]  FilterDiffOutCoefMin=[]  FilterDiffOutCoefMax=[]  SumDenOutMin=[]  SumDenOutMax=[]  SumNumOutMin=[]  SumNumOutMax=[]  ReciprocalOutMin=[]  ReciprocalOutMax=[]  DivideOutMin=[]  DivideOutMax=[]  TunerSelectOption=Transfer Function Based (PID Tuner App)
  cfblk4 : DiscreteTransferFcn
  cfblk5 : simulink/Continuous/PID Controller  Controller=PID  TimeDomain=Discrete-time  SampleTime=-1  IntegratorMethod=Forward Euler  FilterMethod=Forward Euler  Form=Parallel  UseFilter=on  ControllerParametersSource=internal  P=1  I=1  D=0  N=100  InitialConditionSource=internal  InitialConditionForIntegrator=0  InitialConditionForFilter=0  ExternalReset=none  LimitOutput=off  UpperSaturationLimit=inf  LowerSaturationLimit=-inf  LinearizeAsGain=off  AntiWindupMode=none  Kb=1  TrackingMode=off  Kt=1  PParamMin=[]  PParamMax=[]  IParamMin=[]  IParamMax=[]  DParamMin=[]  DParamMax=[]  NParamMin=[]  NParamMax=[]  KbParamMin=[]  KbParamMax=[]  KtParamMin=[]  KtParamMax=[]  POutMin=[]  POutMax=[]  IOutMin=[]  IOutMax=[]  DOutMin=[]  DOutMax=[]  NOutMin=[]  NOutMax=[]  KbOutMin=[]  KbOutMax=[]  KtOutMin=[]  KtOutMax=[]  IntegratorOutMin=[]  IntegratorOutMax=[]  FilterOutMin=[]  FilterOutMax=[]  SumOutMin=[]  SumOutMax=[]  SumI1OutMin=[]  SumI1OutMax=[]  SumI2OutMin=[]  SumI2OutMax=[]  SumI3OutMin=[]  SumI3OutMax=[]  SumDOutMin=[]  SumDOutMax=[]  SaturationOutMin=[]  SaturationOutMax=[]  IntegratorContinuousStateAttributes=''  IntegratorStateMustResolveToSignalObject=off  IntegratorRTWStateStorageClass=Auto  FilterContinuousStateAttributes=''  FilterStateMustResolveToSignalObject=off  FilterRTWStateStorageClass=Auto  DifferentiatorICPrevScaledInput=0  DifferentiatorOutMin=[]  DifferentiatorOutMax=[]  FilterDiffOutCoefMin=[]  FilterDiffOutCoefMax=[]  SumDenOutMin=[]  SumDenOutMax=[]  SumNumOutMin=[]  SumNumOutMax=[]  ReciprocalOutMin=[]  ReciprocalOutMax=[]  DivideOutMin=[]  DivideOutMax=[]  TunerSelectOption=Transfer Function Based (PID Tuner App)
  cfblk6 : Constant  Value=[-338616329.397534]  SampleTime=1
  cfblk7 : Subsystem
  cfblk8 : Subsystem
  cfblk9 : Subsystem
  cfblk2 : Outport
  cfblk14 : Outport  Port=2
  wires:
  cfblk5/1 -> cfblk9/1(cfblk1)
  cfblk11/1 -> cfblk14/1
  cfblk8/1(cfblk2) -> cfblk4/1
  cfblk4/1 -> cfblk2/1
  cfblk6/1 -> cfblk10/1(cfblk1)
  cfblk12/1 -> cfblk3/1
  cfblk7/1(cfblk2) -> cfblk8/1(cfblk1)
  cfblk1/1 -> cfblk5/1
  cfblk3/1 -> cfblk7/1(cfblk1)

== system sampleModel56/cfblk156 ==
  cfblk1 : Inport
  cfblk13 : Inport  Port=2
  Action Port : ActionPort  ActionType=else
  cfblk10 : Subsystem
  cfblk11 : Subsystem
  cfblk12 : Subsystem
  cfblk3 : DiscreteStateSpace  SampleTime=-1
  cfblk4 : DiscreteFir
  cfblk5 : Delay
  cfblk6 : simulink/Discrete/Tapped Delay  vinit=0.0  samptime=-1  NumDelays=1  DelayOrder=Oldest  includeCurrent=off
  cfblk7 : Rounding
  cfblk8 : Math  Operator=log  SaturateOnIntegerOverflow=on
  cfblk9 : Subsystem
  cfblk2 : Outport
  cfblk14 : Outport  Port=2
  wires:
  cfblk7/1 -> cfblk10/1(cfblk1)
  cfblk1/1 -> cfblk7/1
  cfblk9/1(cfblk2) -> cfblk5/1
  cfblk3/1 -> cfblk11/1(cfblk1)
  cfblk4/1 -> cfblk12/1(cfblk1)
  cfblk8/1 -> cfblk2/1
  cfblk6/1 -> cfblk8/1
  cfblk13/1 -> cfblk14/1
  cfblk5/1 -> cfblk4/1
  cfblk11/1(cfblk2) -> cfblk6/1
  cfblk12/1(cfblk2) -> cfblk3/1
  cfblk10/1(cfblk2) -> cfblk9/1(cfblk1)

== system sampleModel56/cfblk157 ==
  cfblk1 : Inport
  Action Port : ActionPort  ActionType=then
  cfblk3 : DiscreteIntegrator  SampleTime=-1  ICPrevOutput=DiscIntNeverNeededParam  ICPrevScaledInput=DiscIntNeverNeededParam
  cfblk4 : Delay  DelayLengthSource=Input port
      settings: InputPortMap=u0,p1
  cfblk5 : simulink/Math Operations/Slider Gain  gain=1  low=0  high=2
  cfblk6 : ComplexToRealImag
  cfblk7 : Subsystem
  cfblk8 : Subsystem
  cfblk9 : Delay
  cfblk2 : Outport
  wires:
  cfblk8/1(cfblk2) -> cfblk4/1
  cfblk1/1 -> cfblk8/1(cfblk1)
  cfblk4/1 -> cfblk5/1
  cfblk6/1 -> cfblk2/1
  cfblk6/2 -> cfblk7/1(cfblk1)
  cfblk5/1 -> cfblk3/1
  cfblk3/1 -> cfblk6/1
  cfblk7/1(cfblk2) -> cfblk9/1
  cfblk9/1 -> cfblk4/2

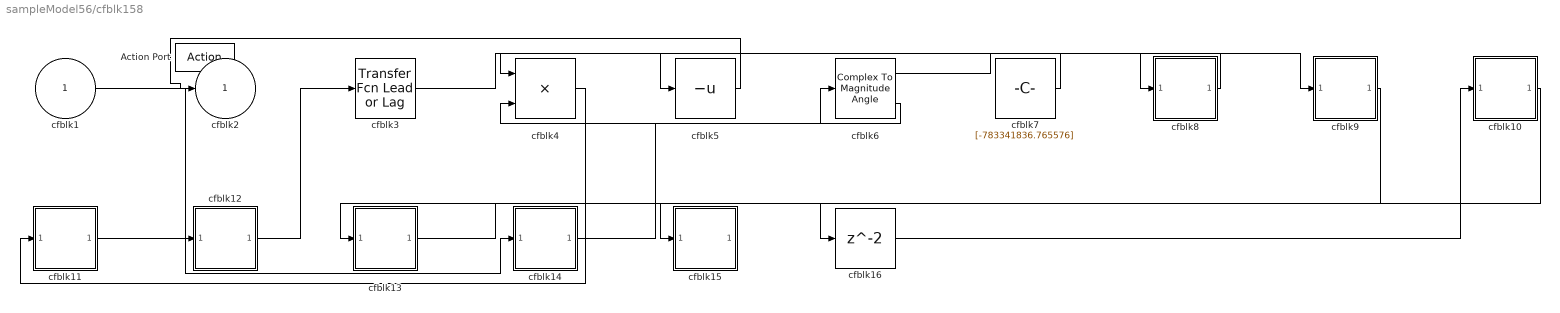
== system sampleModel56/cfblk158 ==
  cfblk1 : Inport
  Action Port : ActionPort  ActionType=else
  cfblk10 : Subsystem
  cfblk11 : Subsystem
  cfblk12 : Subsystem
  cfblk13 : Subsystem
  cfblk14 : Subsystem
  cfblk15 : Subsystem
  cfblk16 : Delay
  cfblk3 : simulink/Discrete/Transfer Fcn Lead or Lag  PoleZ=0.95  ZeroZ=0.75  ICPrevOutput=0.0  ICPrevInput=0.0  DoSatur=off
      settings: SourceProductName=Simulink  SourceProductBaseCode=SL
  cfblk4 : Product  Inputs=**
  cfblk5 : UnaryMinus
  cfblk6 : ComplexToMagnitudeAngle
  cfblk7 : Constant  Value=[-783341836.765576]  SampleTime=1
  cfblk8 : Subsystem
  cfblk9 : Subsystem
  cfblk2 : Outport
  wires:
  cfblk9/1(cfblk2) -> cfblk15/1(cfblk1)
  cfblk12/1(cfblk2) -> cfblk3/1
  cfblk1/1 -> cfblk14/1(cfblk1)
  cfblk5/1 -> cfblk2/1
  cfblk4/1 -> cfblk11/1(cfblk1)
  cfblk14/1(cfblk2) -> cfblk6/1
  cfblk8/1(cfblk2) -> cfblk5/1
  cfblk10/1(cfblk2) -> cfblk13/1(cfblk1)
  cfblk11/1(cfblk2) -> cfblk12/1(cfblk1)
  cfblk7/1 -> cfblk4/1
  cfblk6/1 -> cfblk8/1(cfblk1)
  cfblk6/2 -> cfblk4/2
  cfblk3/1 -> cfblk9/1(cfblk1)
  cfblk13/1(cfblk2) -> cfblk16/1
  cfblk16/1 -> cfblk10/1(cfblk1)

== system sampleModel56/cfblk94 ==
  cfblk1 : Inport
  cfblk2 : Outport
  wires:
  cfblk1/1 -> cfblk2/1

== system sampleModel56/cfblk95 ==
  cfblk1 : Inport
  cfblk2 : Outport
  wires:
  cfblk1/1 -> cfblk2/1

== system sampleModel56/cfblk96 ==
  cfblk1 : Inport
  cfblk2 : Outport
  wires:
  cfblk1/1 -> cfblk2/1

== system sampleModel56/cfblk97 ==
  cfblk1 : Inport
  cfblk2 : Outport
  wires:
  cfblk1/1 -> cfblk2/1

== system sampleModel56/cfblk98 ==
  cfblk1 : Inport
  cfblk2 : Outport
  wires:
  cfblk1/1 -> cfblk2/1

== system sampleModel56/cfblk99 ==
  cfblk1 : Inport
  cfblk2 : Outport
  wires:
  cfblk1/1 -> cfblk2/1

== system sampleModel56/cfblk144/cfblk12 ==
  cfblk1 : Inport
  cfblk2 : Outport
  wires:
  cfblk1/1 -> cfblk2/1

== system sampleModel56/cfblk145/cfblk10 ==
  cfblk1 : Inport
  cfblk2 : Outport
  wires:
  cfblk1/1 -> cfblk2/1

== system sampleModel56/cfblk145/cfblk11 ==
  cfblk1 : Inport
  cfblk2 : Outport
  wires:
  cfblk1/1 -> cfblk2/1

== system sampleModel56/cfblk145/cfblk12 ==
  cfblk1 : Inport
  cfblk2 : Outport
  wires:
  cfblk1/1 -> cfblk2/1

== system sampleModel56/cfblk145/cfblk13 ==
  cfblk1 : Inport
  cfblk2 : Outport
  wires:
  cfblk1/1 -> cfblk2/1

== system sampleModel56/cfblk145/cfblk14 ==
  cfblk1 : Inport
  cfblk2 : Outport
  wires:
  cfblk1/1 -> cfblk2/1

== system sampleModel56/cfblk145/cfblk15 ==
  cfblk1 : Inport
  cfblk2 : Outport
  wires:
  cfblk1/1 -> cfblk2/1

== system sampleModel56/cfblk146/cfblk4 ==
  cfblk1 : Inport
  cfblk2 : Outport
  wires:
  cfblk1/1 -> cfblk2/1
